simulink model "lab3_q"  (R2013b)
settings: Solver=ode45  SolverMode=SingleTasking  StartTime=0.0  StopTime=t_max  RelTol=1e-3
undefined symbols (not defined in the file): k, k2, Lo, Mo, t0, y0
settings Model: CovMetricSettings=dwe  CovHtmlReporting=off  covSaveCumulativeToWorkspaceVar=off  CovSaveSingleToWorkspaceVar=off  CovExternalEMLEnable=on  Creator=lev  LastModifiedBy=lev
settings DataIOCC: LimitDataPoints=off  SaveFormat=StructureWithTime
settings DebuggingCC: UnderspecifiedInitializationDetection=Simplified  MergeDetectMultiDrivingBlocksExec=error  SolverPrmCheckMsg=none  FrameProcessingCompatibilityMsg=error  SFUnexpectedBacktrackingDiag=error  SFNoUnconditionalDefaultTransitionDiag=error
settings HardwareCC: ProdBitPerPointer=64  ProdLargestAtomicFloat=Float  ProdIntDivRoundTo=Zero  ProdEndianess=LittleEndian  ProdHWDeviceType=Specified
settings ModelReferenceCC: PropagateSignalLabelsOutOfModel=on
settings SFSimCC: SimUseLocalCustomCode=on
settings RTWCC: RTWUseLocalCustomCode=on
settings GRTTargetCC: CodeReplacementLibrary=C99 (ISO)  GeneratePreprocessorConditionals=Use local settings

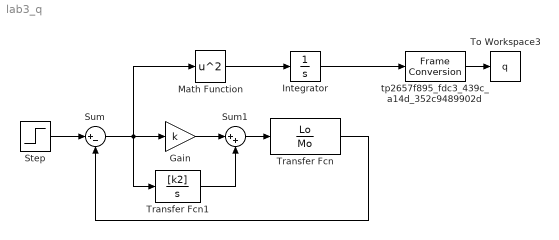
== system lab3_q ==
  Gain : Gain  Gain=k
  Integrator : Integrator
  Math Function : Math  Operator=square  SaturateOnIntegerOverflow=on
  Step : Step  Time=t0  After=y0  SampleTime=0
  Sum : Sum  Inputs=|+-
  Sum1 : Sum  Inputs=|++
  To Workspace3 : ToWorkspace  VariableName=q  SampleTime=-1
      settings: MaxDataPoints=1
  Transfer Fcn : TransferFcn  Numerator=Lo  Denominator=Mo
  Transfer Fcn1 : TransferFcn  Numerator=[k2]  Denominator=[1 0]
  tp2657f895_fdc3_439c_a14d_352c9489902d : FrameConversion  OutFrame=Sample-based
  wires:
  Transfer Fcn/1 -> Sum/2
  Sum/1 -> Math Function/1, Transfer Fcn1/1, Gain/1
  Step/1 -> Sum/1
  Sum1/1 -> Transfer Fcn/1
  Transfer Fcn1/1 -> Sum1/2
  Gain/1 -> Sum1/1
  Math Function/1 -> Integrator/1
  Integrator/1 -> tp2657f895_fdc3_439c_a14d_352c9489902d/1
  tp2657f895_fdc3_439c_a14d_352c9489902d/1 -> To Workspace3/1
